simulink model "ex6_2a1"  (Simulink 7.5)
settings: Solver=ode45  StartTime=0.0  StopTime=0.025  RelTol=1e-3
libraries: powerlib x15, powerlib_extras x1
settings Model: Creator=107108103  LastModifiedBy=Sambhav
settings OptimizationCC: InitFltsAndDblsToZero=on
settings DebuggingCC: StrictBusMsg=Warning

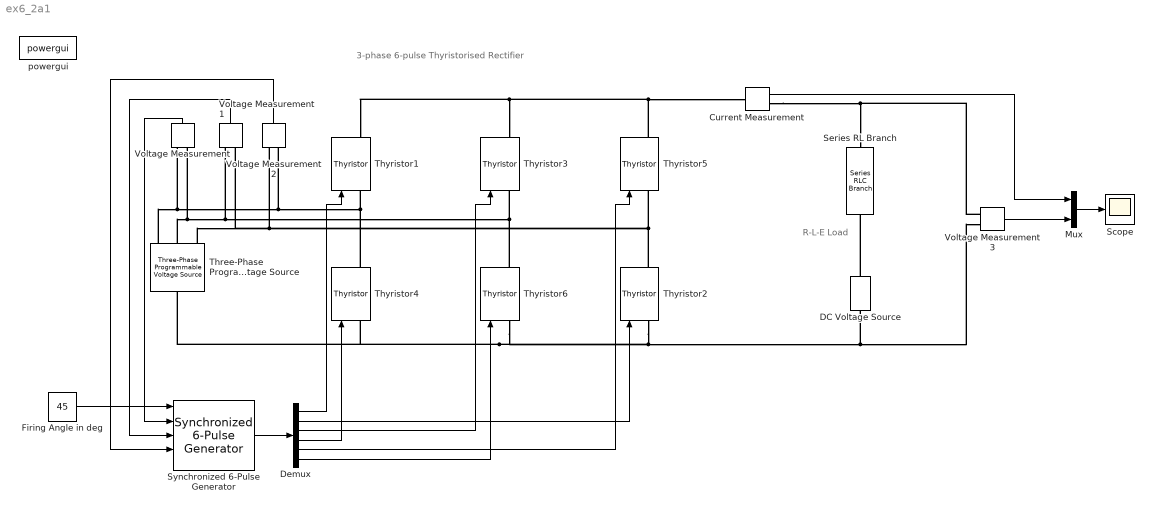
== system ex6_2a1 ==
  note: R-L-E Load
  note: 3-phase 6-pulse Thyristorised Rectifier
  Current Measurement : powerlib/Measurements/Current Measurement  DialogController=POWERSYS.PowerSysDialog  SystemSampleTime=-1  PhasorSimulation=off  OutputType=Complex  PSBequivalent=0
  DC Voltage Source : powerlib/Electrical Sources/DC Voltage Source  DialogController=POWERSYS.PowerSysDialog  SystemSampleTime=-1  Amplitude=100  Measurements=None
  Demux : Demux  Outputs=6
  Firing Angle in deg : Constant  Value=45  OutDataType=sfix(16)  OutScaling=2^0
  Mux : Mux  Inputs=2
  Scope : Scope
  Series RL Branch : powerlib/Elements/Series RLC Branch  DialogController=POWERSYS.PowerSysDialog  PhysicalDomain=powersysdomain  SubClassName=unknown  LeftPortType=p1  RightPortType=p1  LConnTagsString=__new0  RConnTagsString=__new0  BranchType=RL  Resistance=1  Inductance=1e-3  SetiL0=off  InitialCurrent=0  Capacitance=1.0  Setx0=off  InitialVoltage=0  Measurements=None
  Synchronized 6-Pulse Generator : powerlib_extras/Control  Blocks/Synchronized 6-Pulse Generator  DialogController=POWERSYS.PowerSysDialog  SystemSampleTime=-1  freq=60  pwidth=5  Double_Pulse=off
  Three-Phase Programmable Voltage Source : powerlib/Electrical Sources/Three-Phase Programmable Voltage Source  DialogController=POWERSYS.PowerSysDialog  SystemSampleTime=-1  PositiveSequence="[415  0 60]"  VariationEntity=None  VariationType=Step  VariationStep=0.5  VariationRate=10  VariationMagnitude=0.3  VariationFrequency=2  VariationTiming=[1 2]  VariationPhaseA=off  Amplitudes=[1 0.8 1.2 1.0]  TimeValues=[0 0.1 0.15 0.2]  HarmonicGeneration=off  HarmonicA=[3 0.2 -25 0]  HarmonicB=[2 0.15 35 2]  Timing="[0.05  3]"
  Thyristor{1..6} (6 alike) : powerlib/Power Electronics/Thyristor  DialogController=POWERSYS.PowerSysDialog  SystemSampleTime=-1  Ron=0.001  Lon=0  Vf=0.8  IC=0  Rs=500  Cs=250e-9  Measurements=on
  Voltage Measurement{,1..3} (4 alike) : powerlib/Measurements/Voltage Measurement  DialogController=POWERSYS.PowerSysDialog  SystemSampleTime=-1  PhasorSimulation=off  OutputType=Complex  PSBequivalent=0
  powergui : powerlib/powergui  SystemSampleTime=-1  SimulationMode=Continuous  SampleTime=50e-6  frequency=60  SPID=off  DisableSnubberDevices=off  DisableRonSwitches=off  DisableVfSwitches=off  SwTol=0  Interpol=off  frequencyindice=60  echomessages=off  HookPort=off  DisplayEquations=off  FunctionMessages=off  EnableUseOfTLC=off  x0status=blocks  RestoreLinks=warning  ResistiveCurrentMeasurement=off  Frange=[0:2:500]  Ylog=off  Xlog=on  ShowGrid=off  save=off  variable=ZData  ZoomFFT=on  StartTime=0.0  cycles=1  DisplayStyle=1  fundamental=60  FreqAxis=off  MaxFrequency=1000  frequencyindicesteady=1  RmsSteady=1  display=off  Ts=0  methode=off
  wires:
  Synchronized 6-Pulse Generator/1 -> Demux/1
  Firing Angle in deg/1 -> Synchronized 6-Pulse Generator/1
  Voltage Measurement/1 -> Synchronized 6-Pulse Generator/2
  Voltage Measurement1/1 -> Synchronized 6-Pulse Generator/3
  Voltage Measurement2/1 -> Synchronized 6-Pulse Generator/4
  Demux/1 -> Thyristor1/1
  Demux/2 -> Thyristor2/1
  Demux/3 -> Thyristor3/1
  Demux/4 -> Thyristor4/1
  Demux/5 -> Thyristor5/1
  Demux/6 -> Thyristor6/1
  Mux/1 -> Scope/1
  Current Measurement/1 -> Mux/1
  Voltage Measurement3/1 -> Mux/2
  connections:
  Three-Phase Programmable Voltage Source/RConn1 -- Thyristor4/RConn1 -- Thyristor1/LConn1 -- Voltage Measurement2/LConn2 -- Voltage Measurement/LConn1
  Three-Phase Programmable Voltage Source/RConn2 -- Thyristor3/LConn1 -- Thyristor6/RConn1 -- Voltage Measurement1/LConn1 -- Voltage Measurement/LConn2
  Thyristor2/RConn1 -- Three-Phase Programmable Voltage Source/RConn3 -- Voltage Measurement1/LConn2 -- Voltage Measurement2/LConn1 -- Thyristor5/LConn1
  Voltage Measurement3/LConn1 -- Series RL Branch/LConn1 -- Current Measurement/RConn1
  Thyristor2/LConn1 -- Three-Phase Programmable Voltage Source/LConn1 -- Thyristor4/LConn1 -- Thyristor6/LConn1 -- DC Voltage Source/LConn1 -- Voltage Measurement3/LConn2
  DC Voltage Source/RConn1 -- Series RL Branch/RConn1
  Thyristor5/RConn1 -- Thyristor1/RConn1 -- Thyristor3/RConn1 -- Current Measurement/LConn1
